simulink model "Copy_of_PID_control"  (R2025a)
settings: Solver=FixedStepAuto  StartTime=0.0  StopTime=150  FixedStep=0.01  RelTol=1e-3
InitFcn:
  | parameters
values from neighbouring files (symbols this model uses):
  A = pi*(d/2)^2    (= 0.00321699087728)    [parameters.m]    (also in simulations_code.m = 0.00785398163397; test.m = 0.00785398163397)
  A_cross = 0.090    (= 0.09)    [parameters.m]    (also in simulations_code.m = 0.07; test.m = 0.07)
  C_d = 0.136    [parameters.m]    (also in simulations_code.m = 1; test.m = 1)
  constant_amplitude = 0    [Mission.m]    (also in sensitivity.m)
  d1 = 2    [parameters.m]    (also in simulation_matlab.m = 5; simulations_code.m = 5; test.m = 5)
  disturbance_start_time = 120    [compare_controllers.m]    (also in sensitivity.m = 0)
  F_pos = 0.300 * g + m*g    (= 49.70727)    [parameters.m]    (also in sensitivity.m = 0.300 * g + m_values(i)*g; simulation_matlab.m = 2.94; simulations_code.m = 32.37; test.m = 32.37)
  g = 9.81    [parameters.m]    (also in simulation_matlab.m; simulations_code.m; test.m)
  I_hold = 0    [parameters.m]
  I_move = 1.5    [parameters.m]
  m = 4.567+0.2    (= 4.767)    [parameters.m]    (also in simulation_matlab.m = 3; simulations_code.m = 3; test.m = 3)
  p = 0.002    [parameters.m]    (also in simulation_matlab.m; simulations_code.m; test.m)
  p_atm = 101325    [parameters.m]
  rho = 1000    [parameters.m]    (also in simulation_matlab.m; simulations_code.m; test.m)
  rpm_max = 150    [parameters.m]
  sine_amplitude = 0    [Mission.m]    (also in sensitivity.m)
  sine_frequency = 0.05    [Mission.m]    (also in sensitivity.m)
  V_air = 1000e-6    (= 0.001)    [parameters.m]
  V_supply = 11.1    [parameters.m]
  x_max = V_max / A    (= 0.155424749113)    [parameters.m]    (also in simulations_code.m = 0.0636619772368)
libraries: slpidlib x1
settings Model: Creator=hannasennero  LastModifiedBy=hannasennero
settings SolverCC: ZeroCrossAlgorithm=Adaptive
settings DebuggingCC: IgnoredZcDiagnostic=none

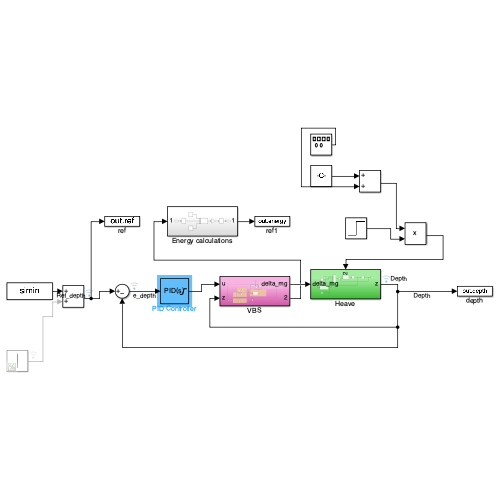
[thumbnail: Simulink's stored preview of the top-level diagram]
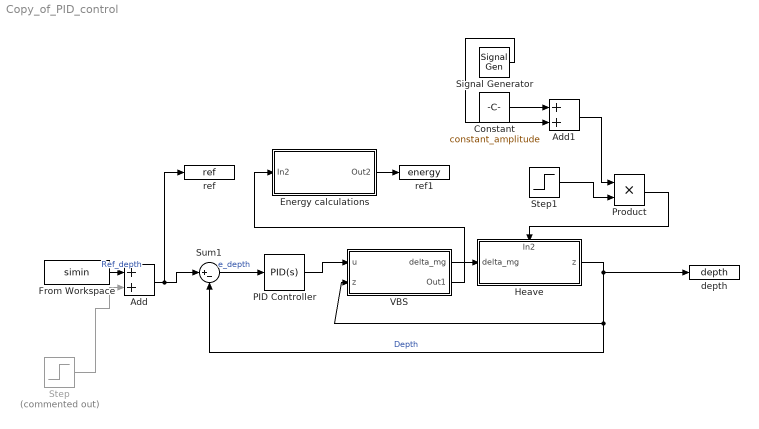
== system Copy_of_PID_control ==
  Add : Sum
  Add1 : Sum
  Constant : Constant  Value=constant_amplitude
  Energy calculations : Subsystem
  From Workspace : FromWorkspace  VariableName=simin
  Heave : Subsystem
      settings: PortSchema="{\"entries\":[{\"content\":{\"sides\":[{\"content\":{\"connectorIds\":[\"In1\"]},\"type\":\"ConnectorPlacement.EquallySpacedRectSide\",\"uuid\":\"6f6a1a60-77e6-4781-930b-afddbe975a8d\"},{\"content\":{\"connectorIds\":[\"Out1\"],\"side\":\"RIGHT\"},\"type\":\"ConnectorPlacement.EquallySpacedRectSide\",\"uuid\":\"4976a1b4-b4d2-4f2a-94be-bdc8db839add\"},{\"content\":{\"connectorIds\":[\"In2\"],\"side\":\"TOP\"},\"type\":\"ConnectorPlacement.EquallySpacedRectSide\",\"uuid\":\"504c6e21-38d1-42a8-8b7b-eda0c51b3613\"}]},\"type\":\"ConnectorPlacement.EquallySpacedConnector\",\"uuid\":\"116e8cad-2b5c-4ef7-8338-d893e08918e3\"}],\"packageUris\":[\"http://schema.mathworks.com/mf0/Connector/R2020b\"],\"version\":\"1.0\"}"
  PID Controller : slpidlib/PID Controller  Controller=PID  Form=Parallel  TimeDomain=Continuous-time  UseExternalTs=off  SampleTime=-1  IntegratorMethod=Forward Euler  FilterMethod=Forward Euler  ControllerParametersSource=internal  P=0.2  I=0  UseKiTs=off  D=3.7  UseExternalDerivativeSource=off  N=10  UseFilter=on  TunerSelectOption=Frequency Response Based  InitialConditionSource=internal  InitialConditionForIntegrator=0  InitialConditionForFilter=0  DifferentiatorICPrevScaledInput=0  ExternalReset=none  TrackingMode=off  Kt=1  LimitOutput=on  SatLimitsSource=internal  UpperSaturationLimit=1  LowerSaturationLimit=-1  LinearizeAsGain=off  AntiWindupMode=none  Kb=1  LimitIntegrator=off  UpperIntegratorSaturationLimit=inf  LowerIntegratorSaturationLimit=-inf  POutMin=[]  POutMax=[]  IOutMin=[]  IOutMax=[]  DOutMin=[]  DOutMax=[]  NOutMin=[]  NOutMax=[]  SumOutMin=[]  SumOutMax=[]  SaturationOutMin=[]  SaturationOutMax=[]  PParamMin=[]  PParamMax=[]  IParamMin=[]  IParamMax=[]  DParamMin=[]  DParamMax=[]  NParamMin=[]  NParamMax=[]  KbParamMin=[]  KbParamMax=[]  KtParamMin=[]  KtParamMax=[]  KbOutMin=[]  KbOutMax=[]  KtOutMin=[]  KtOutMax=[]  IntegratorOutMin=[]  IntegratorOutMax=[]  FilterOutMin=[]  FilterOutMax=[]  SumI1OutMin=[]  SumI1OutMax=[]  SumI2OutMin=[]  SumI2OutMax=[]  SumI3OutMin=[]  SumI3OutMax=[]  SumI4OutMin=[]  SumI4OutMax=[]  SumDOutMin=[]  SumDOutMax=[]  DifferentiatorOutMin=[]  DifferentiatorOutMax=[]  FilterDiffOutCoefMin=[]  FilterDiffOutCoefMax=[]  ReciprocalOutMin=[]  ReciprocalOutMax=[]  SumDenOutMin=[]  SumDenOutMax=[]  SumNumOutMin=[]  SumNumOutMax=[]  DivideOutMin=[]  DivideOutMax=[]  UdiffTsProdOutMin=[]  UdiffTsProdOutMax=[]  NTsProdOutMin=[]  NTsProdOutMax=[]  UintegralTsProdOutMin=[]  UintegralTsProdOutMax=[]  UngainTsProdOutMin=[]  UngainTsProdOutMax=[]  ClampingZeroOutDataTypeStr=Inherit: Inherit via back propagation  ClampingZeroOutMin=[]  ClampingZeroOutMax=[]  FilterDenConstantOutDataTypeStr=Inherit: Inherit via back propagation  FilterDenConstantOutMin=[]  FilterDenConstantOutMax=[]  PCopyOutDataTypeStr=Inherit: Inherit via back propagation  PCopyOutMin=[]  PCopyOutMax=[]  NCopyOutDataTypeStr=Inherit: Inherit via back propagation  NCopyOutMin=[]  NCopyOutMax=[]  IntegratorContinuousStateAttributes=''  IntegratorStateMustResolveToSignalObject=off  IntegratorRTWStateStorageClass=Auto  FilterContinuousStateAttributes=''  FilterStateMustResolveToSignalObject=off  FilterRTWStateStorageClass=Auto  ParallelPVariant=InternalParameters  IdealPVariant=Disabled  IVariant=InternalParameters  DVariant=InternalParameters  IntegratorVariant=Continuous  SatVariant=Enabled  AWVariant=Passthrough  PCopyVariant=Disabled  TRVariant=Disabled  FdbkBlocksVariant=Forward  IdealPFdbkVariant=Disabled  SatFdbkVariant=Disabled  DerivativeFilterVariant=ContFilter  NVariant=InternalParameters  NCopyVariant=Disabled  FilterICVariant=InternalICsFilter  IntegratorICVariant=InternalICs  ExternalResetVariant=Disabled  TRSumVariant=Passthrough  SumFdbkVariant=Disabled  SumVariant=Sum_PID  TsampFilterVariant=InternalTs  TsampNgainVariant=Passthrough  TsampIntegralVariant=Disabled_SignalSpec  ExternalSaturationOutDataTypeStr=Inherit: Same as second input  DerivativeSourceVariant=ErrorSignal  PreIntVariant=InternalPreInt
  Product : Product
  Signal Generator : SignalGenerator  Amplitude=sine_amplitude  Frequency=sine_frequency  Units=rad/sec
  Step : Step  Commented=on  Time=0  SampleTime=0
  Step1 : Step  Time=disturbance_start_time  SampleTime=0
  Sum1 : Sum  Inputs=|+-
  VBS : Subsystem
  depth : ToWorkspace  VariableName=depth  SaveFormat=Timeseries  SampleTime=-1
  ref : ToWorkspace  VariableName=ref  SaveFormat=Timeseries  SampleTime=-1
  ref1 : ToWorkspace  VariableName=energy  SaveFormat=Timeseries  SampleTime=-1
  wires:
  Heave/1(z) -> VBS/2(z), Sum1/2, depth/1  "Depth"
  VBS/1(delta_mg) -> Heave/1(delta_mg)
  Constant/1 -> Add1/1
  Signal Generator/1 -> Add1/2
  Step/1 -> Add/2
  From Workspace/1 -> Add/1  "Ref_depth"
  Add/1 -> ref/1, Sum1/1
  Product/1 -> Heave/2(In2)
  Add1/1 -> Product/1
  Step1/1 -> Product/2
  Sum1/1 -> PID Controller/1  "e_depth"
  PID Controller/1 -> VBS/1(u)
  Energy calculations/1(Out2) -> ref1/1
  VBS/2(Out1) -> Energy calculations/1(In2)

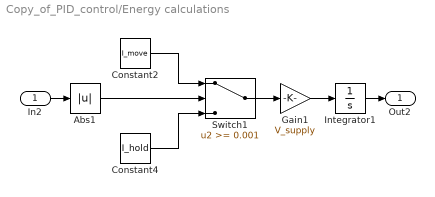
== system Copy_of_PID_control/Energy calculations ==
  In2 : Inport
  Abs1 : Abs  SaturateOnIntegerOverflow=off
  Constant2 : Constant  Value=I_move
  Constant4 : Constant  Value=I_hold
  Gain1 : Gain  Gain=V_supply
  Integrator1 : Integrator
  Switch1 : Switch  Threshold=0.001  SaturateOnIntegerOverflow=off  InputSameDT=off
  Out2 : Outport
  wires:
  In2/1 -> Abs1/1
  Constant4/1 -> Switch1/3
  Switch1/1 -> Gain1/1
  Gain1/1 -> Integrator1/1
  Constant2/1 -> Switch1/1
  Abs1/1 -> Switch1/2
  Integrator1/1 -> Out2/1

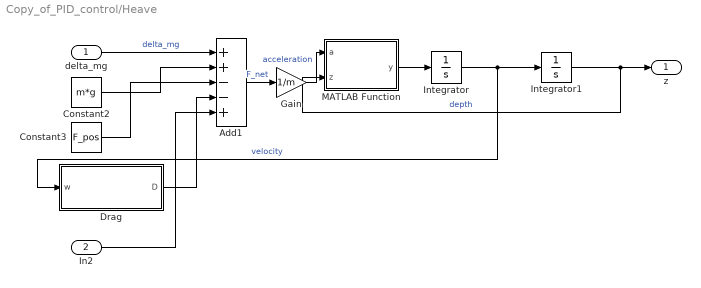
== system Copy_of_PID_control/Heave ==
  delta_mg : Inport
  In2 : Inport  Port=2
  Add1 : Sum  Inputs=++--+
  Constant2 : Constant  Value=m*g
  Constant3 : Constant  Value=F_pos
  Drag : Subsystem
  Gain : Gain  Gain=1/m
  Integrator : Integrator  LowerSaturationLimit=0
  Integrator1 : Integrator  LimitOutput=on  LowerSaturationLimit=0
  MATLAB Function : MATLAB Function  TreatAsAtomicUnit=on
  z : Outport
  wires:
  delta_mg/1 -> Add1/1  "delta_mg"
  Constant2/1 -> Add1/2
  Constant3/1 -> Add1/3
  Add1/1 -> Gain/1  "F_net"
  Integrator/1 -> Drag/1(w), Integrator1/1  "velocity"
  Integrator1/1 -> MATLAB Function/2(z), z/1  "depth"
  MATLAB Function/1(y) -> Integrator/1
  Gain/1 -> MATLAB Function/1(a)  "acceleration"
  In2/1 -> Add1/5
  Drag/1(D) -> Add1/4

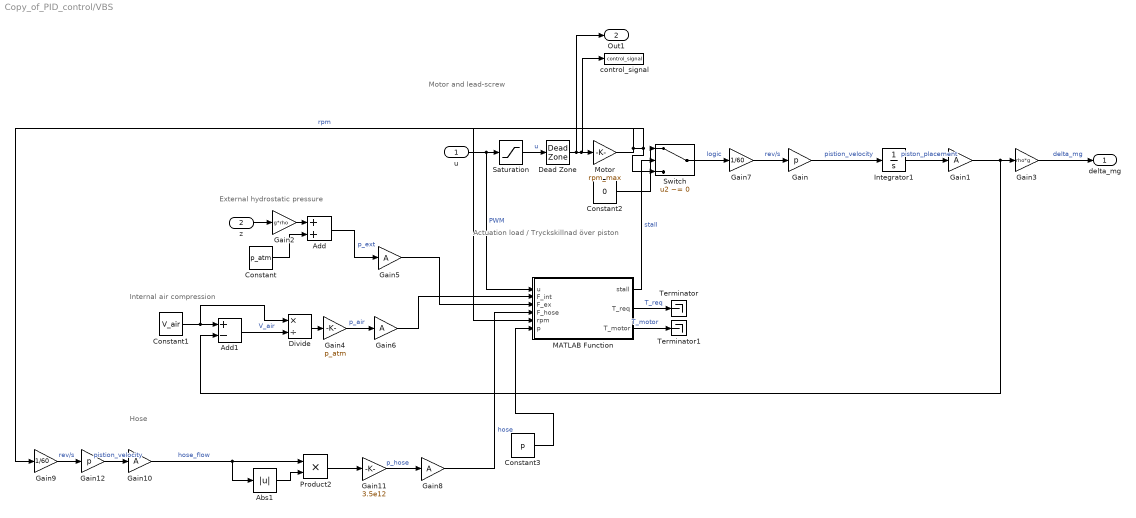
== system Copy_of_PID_control/VBS ==
  note: Motor and lead-screw
  note: External hydrostatic pressure
  note: Internal air compression
  note: Actuation load / Tryckskillnad över piston
  note: Hose
  u : Inport
  z : Inport  Port=2
  Abs1 : Abs  SaturateOnIntegerOverflow=off
  Add : Sum
  Add1 : Sum  Inputs=+-
  Constant : Constant  Value=p_atm
  Constant1 : Constant  Value=V_air
  Constant2 : Constant  Value=0
  Constant3 : Constant  Value=p
  Dead Zone : DeadZone  LowerValue=-0.001  UpperValue=0.001
  Divide : Product  Inputs=*/
  Gain : Gain  Gain=p
  Gain{1,5..6,8,10} (5 alike) : Gain  Gain=A
  Gain11 : Gain  Gain=3.5e12
  Gain12 : Gain  Gain=p
  Gain2 : Gain  Gain=g*rho
  Gain3 : Gain  Gain=rho*g
  Gain4 : Gain  Gain=p_atm
  Gain7 : Gain  Gain=1/60
  Gain9 : Gain  Gain=1/60
  Integrator1 : Integrator  InitialCondition=0.3*g/(A*rho*g)  LimitOutput=on  UpperSaturationLimit=x_max  LowerSaturationLimit=0
  MATLAB Function : MATLAB Function  TreatAsAtomicUnit=on
  Motor : Gain  Gain=rpm_max
  Product2 : Product
  Saturation : Saturate  UpperLimit=1  LowerLimit=-1  LinearizeAsGain=off
  Switch : Switch  Criteria=u2 ~= 0  SaturateOnIntegerOverflow=off  InputSameDT=off
  Terminator : Terminator
  Terminator1 : Terminator
  control_signal : ToWorkspace  VariableName=control_signal  SaveFormat=Timeseries  SampleTime=-1
  delta_mg : Outport
  Out1 : Outport  Port=2
  wires:
  u/1 -> MATLAB Function/1(u), Saturation/1  "PWM"
  Gain/1 -> Integrator1/1  "pistion_velocity"
  Integrator1/1 -> Gain1/1  "piston_placement"
  Gain3/1 -> delta_mg/1  "delta_mg"
  Saturation/1 -> Dead Zone/1  "u"
  z/1 -> Gain2/1
  Gain2/1 -> Add/1
  Constant/1 -> Add/2
  Constant1/1 -> Divide/1, Add1/1
  Gain1/1 -> Add1/2, Gain3/1
  Add1/1 -> Divide/2  "V_air"
  Divide/1 -> Gain4/1
  Gain7/1 -> Gain/1  "rev/s"
  Gain10/1 -> Product2/1, Abs1/1  "hose_flow"
  Product2/1 -> Gain11/1
  Abs1/1 -> Product2/2
  Switch/1 -> Gain7/1  "logic"
  Motor/1 -> Gain9/1, Switch/3, MATLAB Function/5(rpm)  "rpm"
  MATLAB Function/1(stall) -> Switch/2  "stall"
  Add/1 -> Gain5/1  "p_ext"
  Gain4/1 -> Gain6/1  "p_air"
  Gain5/1 -> MATLAB Function/3(F_ex)
  Gain6/1 -> MATLAB Function/2(F_int)
  Gain11/1 -> Gain8/1  "p_hose"
  Gain8/1 -> MATLAB Function/4(F_hose)  "hose"
  Constant3/1 -> MATLAB Function/6(p)
  Gain9/1 -> Gain12/1  "rev/s"
  Gain12/1 -> Gain10/1  "pistion_velocity"
  Constant2/1 -> Switch/1
  MATLAB Function/2(T_req) -> Terminator/1  "T_req"
  MATLAB Function/3(T_motor) -> Terminator1/1  "T_motor"
  Dead Zone/1 -> Out1/1, Motor/1, control_signal/1

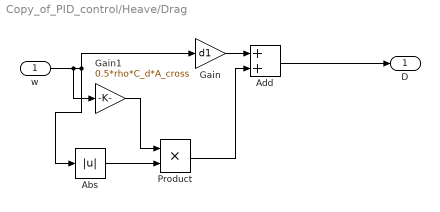
== system Copy_of_PID_control/Heave/Drag ==
  w : Inport
  Abs : Abs  SaturateOnIntegerOverflow=off
  Add : Sum
  Gain : Gain  Gain=d1
  Gain1 : Gain  Gain=0.5*rho*C_d*A_cross
  Product : Product
  D : Outport
  wires:
  w/1 -> Gain/1, Abs/1, Gain1/1
  Gain/1 -> Add/1
  Abs/1 -> Product/2
  Gain1/1 -> Product/1
  Product/1 -> Add/2
  Add/1 -> D/1

== matlab function Copy_of_PID_control/VBS/MATLAB Function ==
  data: u input; stall output; F_int input; F_ex input; F_hose input; rpm input; p input; T_req output; T_motor output
function [stall,T_req,T_motor] = fcn(u,F_int,F_ex,F_hose, rpm,p)
if u > 0
    F_load = F_int-F_ex + F_hose;
else
    F_load = F_ex-F_int+F_hose;
end

%convert p to T
T_req = F_load*p/(2*pi);

T_motor = 0.540 - 0.00029*rpm;

if T_motor <= 0
    stall = 1;
elseif  (T_motor - T_req) < 0
    stall = 1;
else
    stall = 0;
end

== matlab function Copy_of_PID_control/Heave/MATLAB Function ==
  data: a input; y output; z input
function y = fcn(a,z)
if a<= 0 && z <= 0
    y = 0;
else
    y = a;
end
